simulink model "serial"  (R2015a)
settings: Solver=ode45  StartTime=0.0  StopTime=10.0  RelTol=1e-3
libraries: instrumentlib x3
settings Model: Creator=Jose Roldan  LastModifiedBy=Jose Roldan

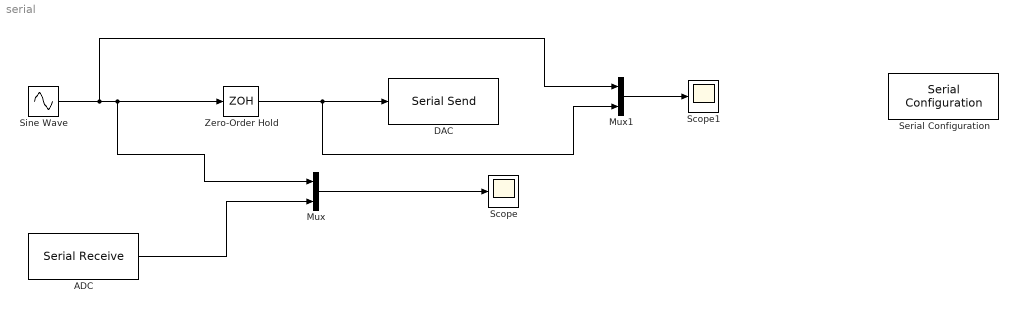
== system serial ==
  ADC : instrumentlib/Serial Receive  ComPortMenu=<Please select a port...>  ComPort=<Please select a port...>  Terminator=<none>  DataSize=[1 1]  DataType=double  EnableBlockingMode=on  ActionDataUnavailable=Output last received value  CustomValue=0  SampleTime=2*0.01
  "DAC " : instrumentlib/Serial Send  ComPortMenu=<Please select a port...>  ComPort=<Please select a port...>  Terminator=<none>  EnableBlockingMode=on
  Mux : Mux  Inputs=2
  Mux1 : Mux  Inputs=2
  Scope : Scope
  Scope1 : Scope
  Serial Configuration : instrumentlib/Serial Configuration  Priority=-200000  ComPortMenu=<Please select a port...>  ComPort=<Please select a port...>  BaudRate=9600  DataBits=8  Parity=none  StopBits=1  FlowControl=none  Timeout=10  ByteOrder=LittleEndian
  Sine Wave : Sin  Amplitude=2  Frequency=1/0.1  SampleTime=0
  Zero-Order Hold : ZeroOrderHold  SampleTime=0.01
  wires:
  Mux/1 -> Scope/1
  Sine Wave/1 -> Mux1/1, Zero-Order Hold/1, Mux/1
  ADC/1 -> Mux/2
  Zero-Order Hold/1 -> Mux1/2, "DAC "/1
  Mux1/1 -> Scope1/1
